simulink model "Simulation_servo_tangage_1_v2_sujet"  (R2016b)
settings: Solver=FixedStepDiscrete  StartTime=0.0  StopTime=inf  RelTol=1e-3  EnableMultiTasking=on
settings Model: Creator=Francois  LastModifiedBy=Xavier
settings DataIOCC: LimitDataPoints=on  SaveFormat=Array  SignalLoggingSaveFormat=ModelDataLogs
settings OptimizationCC: ExpressionDepthLimit=2147483647  LifeSpan=inf
settings DebuggingCC: UnderspecifiedInitializationDetection=Classic  MergeDetectMultiDrivingBlocksExec=none  SolverPrmCheckMsg=warning  FcnCallInpInsideContextMsg=warning  StateNameClashWarn=warning  SFUnexpectedBacktrackingDiag=warning  SFNoUnconditionalDefaultTransitionDiag=warning  SFExecutionAtInitializationDiag=none
settings HardwareCC: ProdBitPerPointer=32  ProdBitPerSizeT=32  ProdBitPerPtrDiffT=32  ProdLargestAtomicFloat=None  ProdIntDivRoundTo=Undefined  ProdEndianess=Unspecified  ProdWordSize=32  ProdHWDeviceType=32-bit Generic
settings ModelReferenceCC: PropagateSignalLabelsOutOfModel=off
settings GRTTargetCC: TargetLangStandard=C89/C90 (ANSI)  GeneratePreprocessorConditionals=Disable all
settings ConfigComp: CovMetricSettings=dw  CovHtmlReporting=on  CovSaveCumulativeToWorkspaceVar=on  CovSaveSingleToWorkspaceVar=on  CovExternalEMLEnable=off

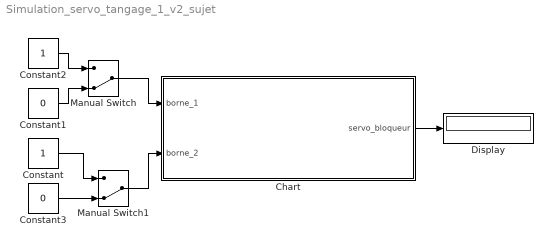
== system Simulation_servo_tangage_1_v2_sujet ==
  Chart : Stateflow chart  TreatAsAtomicUnit=on
  Constant : Constant
  Constant1 : Constant  Value=0
  Constant2 : Constant
  Constant3 : Constant  Value=0
  Display : Display
  Manual Switch : ManualSwitch  CurrentSetting=0
  Manual Switch1 : ManualSwitch  CurrentSetting=0
  wires:
  Manual Switch/1 -> Chart/1(borne_1)
  Manual Switch1/1 -> Chart/2(borne_2)
  Constant2/1 -> Manual Switch/1
  Constant1/1 -> Manual Switch/2
  Constant/1 -> Manual Switch1/1
  Constant3/1 -> Manual Switch1/2
  Chart/1(servo_bloqueur) -> Display/1

== stateflow chart Simulation_servo_tangage_1_v2_sujet/Chart ==
  state tangage_bloque
    during : servo_bloqueur = 45;
  state tangage_limite
    during : servo_bloqueur = 90;
  state tangage_libre
    during : servo_bloqueur = 135;
  (default) -> (junction 15)
  (junction 15) -> tangage_bloque [order 1] : [borne_1==1 && borne_2==1]
  (junction 15) -> tangage_libre [order 3] : [borne_1==1 && borne_2==0]
  (junction 15) -> tangage_limite [order 2]
  tangage_libre -> tangage_limite
  tangage_bloque -> tangage_limite
  tangage_limite -> tangage_libre [order 2]
  tangage_limite -> tangage_bloque [order 1]
  data: borne_1 input; borne_2 input; servo_bloqueur output double
